simulink model "Display_Test"  (R2020a)
settings: Solver=VariableStepAuto  StartTime=0.0  StopTime=inf  RelTol=1e-3
settings Model: Creator=LAB-OREN3  LastModifiedBy=LAB-OREN3
settings DataIOCC: ReturnWorkspaceOutputs=off
settings DebuggingCC: ArithmeticOperatorsInVariantConditions=warning
settings SFSimCC: SimUseLocalCustomCode=off  CustomCodeUndefinedFunction=UseInterfaceOnly
settings RTWCC: RTWUseLocalCustomCode=off
settings CodeAppCC: StateflowObjectComments=on

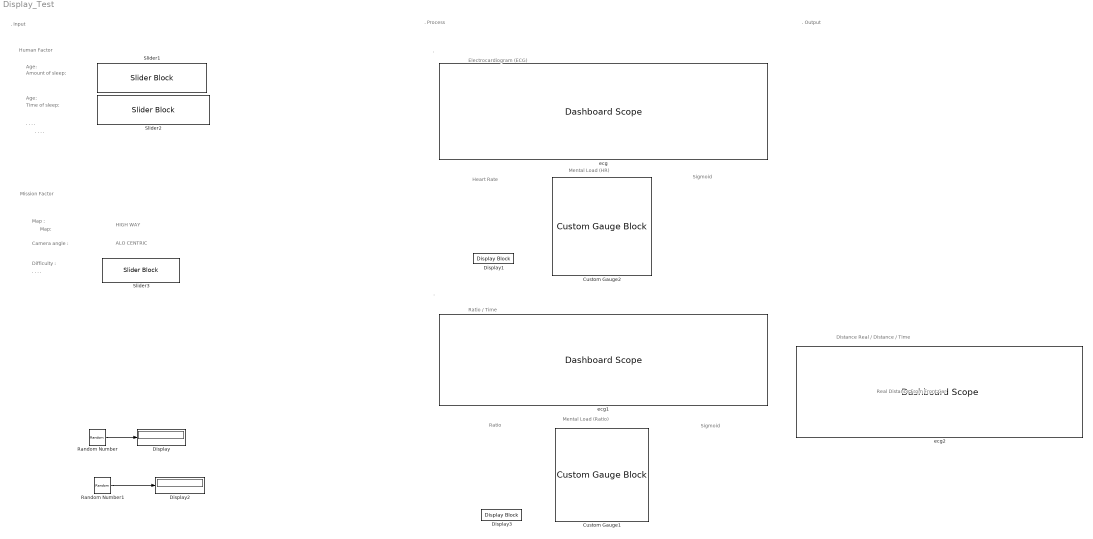
== system Display_Test ==
  note: Electrocardiogram (ECG)
  note: .
      | .
      | .
      | .
  note: .
  note: Heart Rate
  note: Human Factor
  note: Map :
  note: .
      | .
      | .
      | .
  note: .
      | .
      | .
      | .
  note: . Output
  note: . Process
  note: HIGH WAY
  note: Amount of sleep:
  note: . Input
  note: ALO CENTRIC
  note: Real Distance From Front Car
  note: .
  note: Ratio / Time
  note: Ratio
  note: Camera angle :
  note: Age:
  note: Mental Load (HR)
  note: Mental Load (Ratio)
  note: Sigmoid
  note: Difficulty :
  note: Mission Factor
  note: Sigmoid
  note: Distance Real / Distance / Time
  note: Map:
  note: Age:
  note: Time of sleep:
  Custom Gauge1 : CustomGaugeBlock  LabelPosition=Hide  NeedleImage=data:image/svg+xml;base64,PD94bWwgdmVyc2lvbj0iMS4wIiBlbmNvZGluZz0idXRmLTgiPz4KPCEtLSBHZW5lcmF0b3I6IEFkb2JlIElsbHVzdHJhdG9yIDE5LjIuMSwgU1ZHIEV4cG9ydCBQbHVnLUluIC4gU1ZHIFZlcnNpb246IDYuMDAgQnVpbGQgMCkgIC0tPgo8c3ZnIHZlcnNpb249IjEuMSIgeG1sbnM9Imh0dHA6Ly93d3cudzMub3JnLzIwMDAvc3ZnIiB4bWxuczp4bGluaz0iaHR0cDovL3d3dy53My5vcmcvMTk5OS94bGluayIgeD0iMHB4IiB5PSIwcHgiCgkgdmlld0JveD0iMCAwIDIwMCA1MCIgc3R5bGU9ImVuYWJsZS1iYWNrZ3JvdW5kOm5ldyAw ...(+9940 chars)  NeedleXPos=0.3499172390096674  NeedleYPos=0.47640815567113937  NeedleHeight=0.14538535381695605  NeedleWidth=0.23951163488118776  NeedleInitialRotation=-59.94322499147643  BackgroundImage=data:image/svg+xml;base64,PD94bWwgdmVyc2lvbj0iMS4wIiBlbmNvZGluZz0iVVRGLTgiIHN0YW5kYWxvbmU9Im5vIj8+CjwhLS0gR2VuZXJhdG9yOiBBZG9iZSBJbGx1c3RyYXRvciAxOS4yLjEsIFNWRyBFeHBvcnQgUGx1Zy1JbiAuIFNWRyBWZXJzaW9uOiA2LjAwIEJ1aWxkIDApICAtLT4KCjxzdmcKICAgeG1sbnM6ZGM9Imh0dHA6Ly9wdXJsLm9yZy9kYy9lbGVtZW50cy8xLjEvIgogICB4bWxuczpjYz0iaHR0cDovL2NyZWF0aXZlY29tbW9ucy5vcmcvbnMjIgogICB4bWxuczpyZGY9Imh0dHA6Ly93d3cudzMub3JnLzE5OTkvMDIvMjItcmRmLXN5bnRh ...(+9660 chars)  GaugeMax=1  GaugeArcDefined=true  GaugeArcRadius=0.17024022317539744  GaugeArcStrokeWidth=0.049784812900674394  GaugeArcRotation=240.5385250290321  GaugeArcRatio=0.8333333333333  GaugeArcTransparency=0  ValueArcTransparency=0  ValueArcColor=#1759b0  GaugeTickTransparency=0.55  GaugeTickColor=#faf5c8  ScaleColorsJSON="[{\"Min\":0,\"Max\":0.4,\"Color\":[0.39215686274509803,0.83137254901960778,0.074509803921568626]},{\"Min\":0.4,\"Max\":0.7,\"Color\":[0.92941176470588238,0.69411764705882351,0.12549019607843137]},{\"Min\":0.7,\"Max\":1,\"Color\":[0.996078431372549,0.2,0.0392156862745098]}]"  fixedAspectRatio=on  IsLinearGauge=false  GaugeTrackLeft=0.35  GaugeTrackTop=0.35  GaugeTrackHeight=0.1  GaugeTrackWidth=0.3  GaugeTrackRotation=0
  Custom Gauge2 : CustomGaugeBlock  LabelPosition=Hide  NeedleImage=data:image/svg+xml;base64,PD94bWwgdmVyc2lvbj0iMS4wIiBlbmNvZGluZz0idXRmLTgiPz4KPCEtLSBHZW5lcmF0b3I6IEFkb2JlIElsbHVzdHJhdG9yIDE5LjIuMSwgU1ZHIEV4cG9ydCBQbHVnLUluIC4gU1ZHIFZlcnNpb246IDYuMDAgQnVpbGQgMCkgIC0tPgo8c3ZnIHZlcnNpb249IjEuMSIgeG1sbnM9Imh0dHA6Ly93d3cudzMub3JnLzIwMDAvc3ZnIiB4bWxuczp4bGluaz0iaHR0cDovL3d3dy53My5vcmcvMTk5OS94bGluayIgeD0iMHB4IiB5PSIwcHgiCgkgdmlld0JveD0iMCAwIDIwMCA1MCIgc3R5bGU9ImVuYWJsZS1iYWNrZ3JvdW5kOm5ldyAw ...(+9940 chars)  NeedleXPos=0.3499172390096674  NeedleYPos=0.47640815567113937  NeedleHeight=0.14538535381695605  NeedleWidth=0.23951163488118776  NeedleInitialRotation=-59.94322499147643  BackgroundImage=data:image/svg+xml;base64,PD94bWwgdmVyc2lvbj0iMS4wIiBlbmNvZGluZz0iVVRGLTgiIHN0YW5kYWxvbmU9Im5vIj8+CjwhLS0gR2VuZXJhdG9yOiBBZG9iZSBJbGx1c3RyYXRvciAxOS4yLjEsIFNWRyBFeHBvcnQgUGx1Zy1JbiAuIFNWRyBWZXJzaW9uOiA2LjAwIEJ1aWxkIDApICAtLT4KCjxzdmcKICAgeG1sbnM6ZGM9Imh0dHA6Ly9wdXJsLm9yZy9kYy9lbGVtZW50cy8xLjEvIgogICB4bWxuczpjYz0iaHR0cDovL2NyZWF0aXZlY29tbW9ucy5vcmcvbnMjIgogICB4bWxuczpyZGY9Imh0dHA6Ly93d3cudzMub3JnLzE5OTkvMDIvMjItcmRmLXN5bnRh ...(+9660 chars)  GaugeMax=1  GaugeArcDefined=true  GaugeArcRadius=0.17024022317539744  GaugeArcStrokeWidth=0.049784812900674394  GaugeArcRotation=240.5385250290321  GaugeArcRatio=0.8333333333333  GaugeArcTransparency=0  ValueArcTransparency=0  ValueArcColor=#1759b0  GaugeTickColor=#faf5c8  ScaleColorsJSON="[{\"Min\":0,\"Max\":0.4,\"Color\":[0.39215686274509803,0.83137254901960778,0.074509803921568626]},{\"Min\":0.4,\"Max\":0.7,\"Color\":[0.92941176470588238,0.69411764705882351,0.12549019607843137]},{\"Min\":0.7,\"Max\":1,\"Color\":[0.996078431372549,0.2,0.0392156862745098]}]"  IsLinearGauge=false  GaugeTrackLeft=0.35  GaugeTrackTop=0.35  GaugeTrackHeight=0.1  GaugeTrackWidth=0.3  GaugeTrackRotation=0
  Display : Display
  Display1 : DisplayBlock  LabelPosition=Hide  Format=Integer  Transparency=1
  Display2 : Display
  Display3 : DisplayBlock  LabelPosition=Hide  Format=Integer  Transparency=1
  Random Number : RandomNumber  Mean=7  SampleTime=1
  Random Number1 : RandomNumber  Mean=5  SampleTime=1
  Slider1 : SliderBlock  LabelPosition=Hide  ScaleMax=10
  Slider2 : SliderBlock  LabelPosition=Hide  ScaleMin=10  ScaleMax=70  TickInterval=10
  Slider3 : SliderBlock  LabelPosition=Hide  ScaleMin=1  ScaleMax=3  TickInterval=1
  ecg : DashboardScope  Tag=ECG  TimeSpan=100  Ymin=0  Ymax=100000  LegendPosition=Hide  ScaleAtStop=off
  ecg1 : DashboardScope  Tag=ECG  ShowInitialText=off  TimeSpan=100  Ymin=0  Ymax=100000  LegendPosition=Hide  ScaleAtStop=off
  ecg2 : DashboardScope  Tag=ECG  ShowInitialText=off  TimeSpan=100  Ymin=0  Ymax=20  LegendPosition=Hide  ScaleAtStop=off
  wires:
  Random Number/1 -> Display/1
  Random Number1/1 -> Display2/1
